simulink model "ITCG_3D"  (R2023b)
settings: Solver=FixedStepAuto  StartTime=0.0  StopTime=45  FixedStep=1/100  RelTol=1e-3
libraries: simulink x1
settings Model: NumberOfSteps=10  PacingRate=5  Creator=Administrator  LastModifiedBy=lmj04
settings DebuggingCC: UnderSpecifiedDimensionMsg=warning

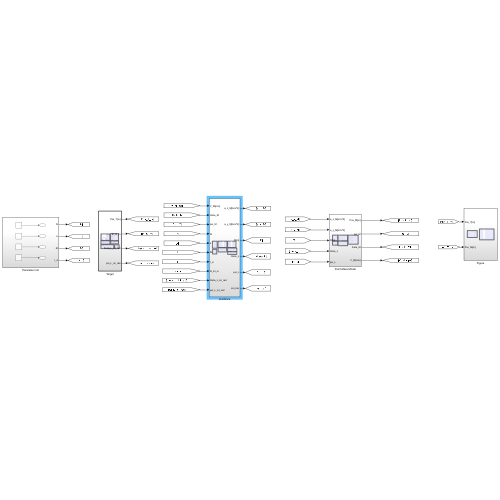
[thumbnail: Simulink's stored preview of the top-level diagram]
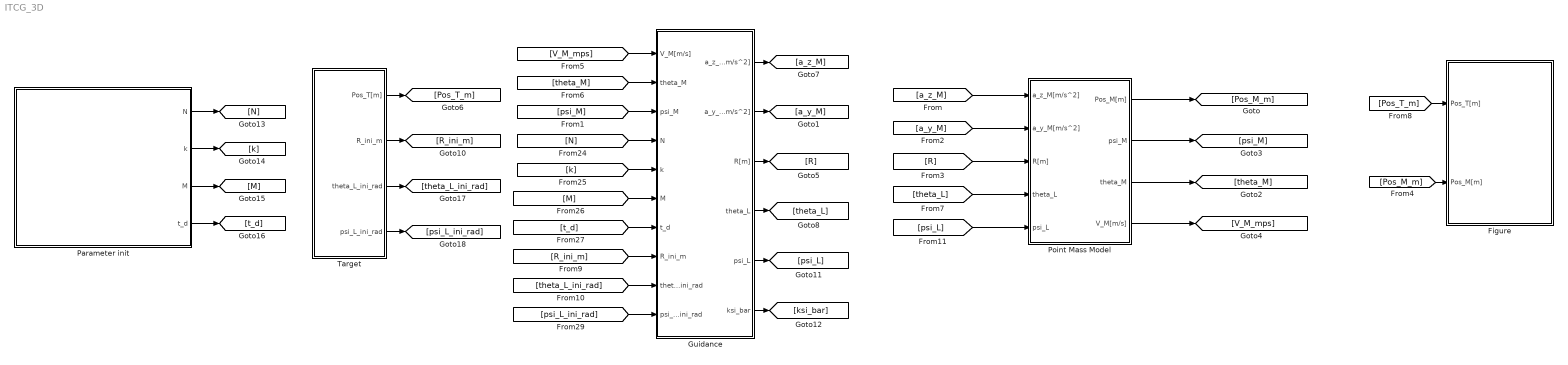
== system ITCG_3D ==
  Figure : Subsystem
  Guidance : Subsystem
  Parameter init : Subsystem
  Point Mass Model : Subsystem
  Target : Subsystem  TreatAsAtomicUnit=on
  wires:
  Target/1(Pos_T[m]) -> [Pos_T_m]
  Guidance/1(a_z_M[m/s^2]) -> [a_z_M]
  [V_M_mps] -> Guidance/1(V_M[m/s])
  Point Mass Model/1(Pos_M[m]) -> [Pos_M_m]
  Point Mass Model/4(V_M[m/s]) -> [V_M_mps]
  Guidance/2(a_y_M[m/s^2]) -> [a_y_M]
  Guidance/3(R[m]) -> [R]
  [R] -> Point Mass Model/3(R[m])
  Guidance/4(theta_L) -> [theta_L]
  [theta_L] -> Point Mass Model/4(theta_L)
  Point Mass Model/2(psi_M) -> [psi_M]
  Point Mass Model/3(theta_M) -> [theta_M]
  [theta_M] -> Guidance/2(theta_M)
  [psi_M] -> Guidance/3(psi_M)
  Guidance/5(psi_L) -> [psi_L]
  [psi_L] -> Point Mass Model/5(psi_L)
  Guidance/6(ksi_bar) -> [ksi_bar]
  Parameter init/2(k) -> [k]
  Parameter init/1(N) -> [N]
  Parameter init/3(M) -> [M]
  Parameter init/4(t_d) -> [t_d]
  [M] -> Guidance/6(M)
  [t_d] -> Guidance/7(t_d)
  [N] -> Guidance/4(N)
  [k] -> Guidance/5(k)
  [a_y_M] -> Point Mass Model/2(a_y_M[m/s^2])
  Target/2(R_ini_m) -> [R_ini_m]
  [R_ini_m] -> Guidance/8(R_ini_m)
  Target/3(theta_L_ini_rad) -> [theta_L_ini_rad]
  Target/4(psi_L_ini_rad) -> [psi_L_ini_rad]
  [theta_L_ini_rad] -> Guidance/9(theta_L_ini_rad)
  [psi_L_ini_rad] -> Guidance/10(psi_L_ini_rad)
  [a_z_M] -> Point Mass Model/1(a_z_M[m/s^2])
  [Pos_M_m] -> Figure/2(Pos_M[m])
  [Pos_T_m] -> Figure/1(Pos_T[m])

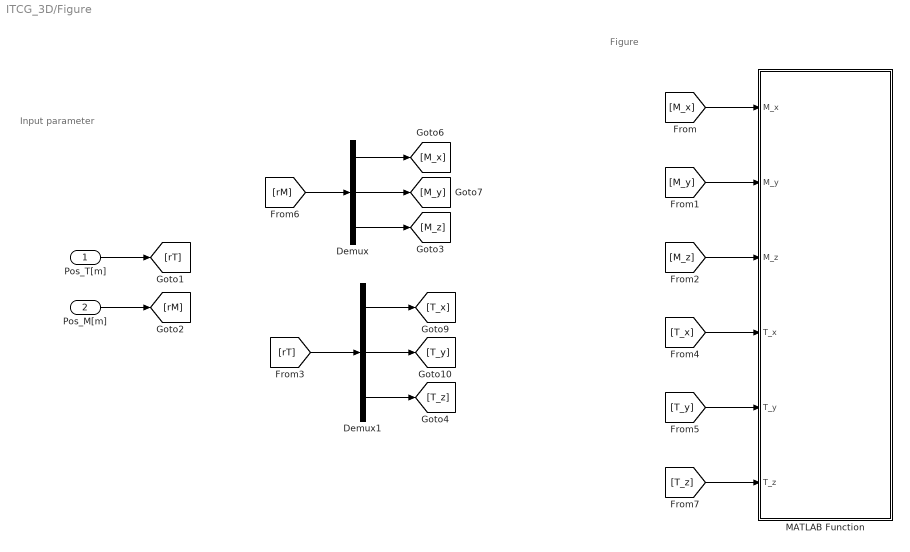
== system ITCG_3D/Figure ==
  note: Figure
  note: Input parameter
  Pos_T[m] : Inport
  Pos_M[m] : Inport  Port=2
  Demux : Demux  Outputs=3
  Demux1 : Demux  Outputs=3
  MATLAB Function : MATLAB Function  TreatAsAtomicUnit=on
  wires:
  Pos_T[m]/1 -> [rT]
  Pos_M[m]/1 -> [rM]
  [rT] -> Demux1/1
  Demux1/1 -> [T_x]
  Demux1/2 -> [T_y]
  Demux/2 -> [M_y]
  Demux/1 -> [M_x]
  Demux/3 -> [M_z]
  Demux1/3 -> [T_z]
  [M_x] -> MATLAB Function/1(M_x)
  [M_y] -> MATLAB Function/2(M_y)
  [M_z] -> MATLAB Function/3(M_z)
  [T_x] -> MATLAB Function/4(T_x)
  [T_y] -> MATLAB Function/5(T_y)
  [T_z] -> MATLAB Function/6(T_z)
  [rM] -> Demux/1

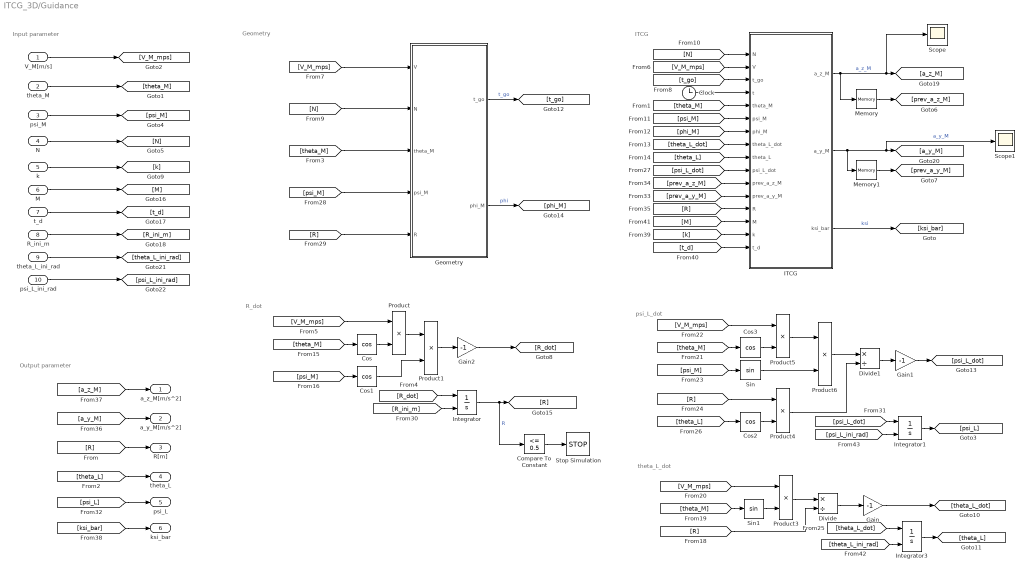
== system ITCG_3D/Guidance ==
  note: ITCG
  note: Geometry
  note: Input parameter
  note: Output parameter
  note: psi_L_dot
  note: theta_L_dot
  note: R_dot
  V_M[m/s] : Inport
  theta_M : Inport  Port=2
  psi_M : Inport  Port=3
  N : Inport  Port=4
  k : Inport  Port=5
  M : Inport  Port=6
  t_d : Inport  Port=7
  R_ini_m : Inport  Port=8
  theta_L_ini_rad : Inport  Port=9
  psi_L_ini_rad : Inport  Port=10
  Clock : Clock
  Compare To Constant : simulink/Logic and Bit Operations/Compare To Constant  relop=<=  const=0.5  OutDataTypeStr=boolean
  Cos{,1..3} (4 alike) : Trigonometry  Operator=cos
  Divide : Product  Inputs=*/
  Divide1 : Product  Inputs=*/
  Gain : Gain  Gain=-1
  Gain1 : Gain  Gain=-1
  Gain2 : Gain  Gain=-1
  Geometry : MATLAB Function  TreatAsAtomicUnit=on
  ITCG : MATLAB Function  TreatAsAtomicUnit=on
  Integrator : Integrator  InitialConditionSource=external  InitialCondition=sqrt(300^2+500^2)
  Integrator1 : Integrator  InitialConditionSource=external
  Integrator3 : Integrator  InitialConditionSource=external
  Memory : Memory
  Memory1 : Memory
  Product{,1,3..6} (6 alike) : Product
  Scope : Scope
  Scope1 : Scope
  Sin : Trigonometry
  Sin1 : Trigonometry
  Stop Simulation : Stop
  a_z_M[m/s^2] : Outport
  a_y_M[m/s^2] : Outport  Port=2
  R[m] : Outport  Port=3
  theta_L : Outport  Port=4
  psi_L : Outport  Port=5
  ksi_bar : Outport  Port=6
  wires:
  V_M[m/s]/1 -> [V_M_mps]
  [V_M_mps] -> Geometry/1(V)
  N/1 -> [N]
  [N] -> Geometry/2(N)
  ITCG/3(ksi_bar) -> [ksi_bar]  "ksi"
  [N] -> ITCG/1(N)
  [V_M_mps] -> ITCG/2(V)
  [t_go] -> ITCG/3(t_go)
  Clock/1 -> ITCG/4(t)
  [theta_M] -> ITCG/5(theta_M)
  [psi_M] -> ITCG/6(psi_M)
  [phi_M] -> ITCG/7(phi_M)
  [theta_L_dot] -> ITCG/8(theta_L_dot)
  [theta_L] -> ITCG/9(theta_L)
  theta_M/1 -> [theta_M]
  psi_M/1 -> [psi_M]
  [V_M_mps] -> Product/1
  Cos/1 -> Product/2
  [theta_M] -> Cos/1
  Product/1 -> Product1/1
  [psi_M] -> Cos1/1
  Cos1/1 -> Product1/2
  Gain2/1 -> [R_dot]
  Sin1/1 -> Product3/2
  [V_M_mps] -> Product3/1
  [theta_M] -> Sin1/1
  Product3/1 -> Divide/1
  [R] -> Divide/2
  Divide/1 -> Gain/1
  [theta_M] -> Cos3/1
  [V_M_mps] -> Product5/1
  Cos3/1 -> Product5/2
  Product5/1 -> Product6/1
  [psi_M] -> Sin/1
  Sin/1 -> Product6/2
  [theta_L_dot] -> Integrator3/1
  Integrator3/1 -> [theta_L]
  Product6/1 -> Divide1/1
  Divide1/1 -> Gain1/1
  Geometry/1(t_go) -> [t_go]  "t_go"
  Geometry/2(phi_M) -> [phi_M]  "phi"
  [theta_M] -> Geometry/3(theta_M)
  [theta_L] -> theta_L/1
  [R] -> R[m]/1
  [psi_M] -> Geometry/4(psi_M)
  [psi_L_dot] -> ITCG/10(psi_L_dot)
  [R_dot] -> Integrator/1
  [a_y_M] -> a_y_M[m/s^2]/1
  [a_z_M] -> a_z_M[m/s^2]/1
  ITCG/1(a_z_M) -> Scope/1, [a_z_M], Memory/1  "a_z_M"
  ITCG/2(a_y_M) -> Memory1/1, Scope1/1, [a_y_M]  "a_y_M"
  Gain/1 -> [theta_L_dot]
  Gain1/1 -> [psi_L_dot]
  Integrator/1 -> [R], Compare To Constant/1  "R"
  [R] -> Product4/1
  Cos2/1 -> Product4/2
  [theta_L] -> Cos2/1
  Product4/1 -> Divide1/2
  Product1/1 -> Gain2/1
  [R] -> Geometry/5(R)
  [psi_L_dot] -> Integrator1/1
  Integrator1/1 -> [psi_L]
  [psi_L] -> psi_L/1
  Memory/1 -> [prev_a_z_M]
  Memory1/1 -> [prev_a_y_M]
  [prev_a_y_M] -> ITCG/12(prev_a_y_M)
  [prev_a_z_M] -> ITCG/11(prev_a_z_M)
  [R] -> ITCG/13(R)
  [ksi_bar] -> ksi_bar/1
  k/1 -> [k]
  M/1 -> [M]
  t_d/1 -> [t_d]
  [M] -> ITCG/14(M)
  [k] -> ITCG/15(k)
  [t_d] -> ITCG/16(t_d)
  Compare To Constant/1 -> Stop Simulation/1
  R_ini_m/1 -> [R_ini_m]
  [R_ini_m] -> Integrator/2
  theta_L_ini_rad/1 -> [theta_L_ini_rad]
  psi_L_ini_rad/1 -> [psi_L_ini_rad]
  [theta_L_ini_rad] -> Integrator3/2
  [psi_L_ini_rad] -> Integrator1/2

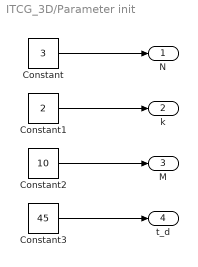
== system ITCG_3D/Parameter init ==
  Constant : Constant  Value=3
  Constant1 : Constant  Value=2
  Constant2 : Constant  Value=10
  Constant3 : Constant  Value=45
  N : Outport
  k : Outport  Port=2
  M : Outport  Port=3
  t_d : Outport  Port=4
  wires:
  Constant/1 -> N/1
  Constant1/1 -> k/1
  Constant2/1 -> M/1
  Constant3/1 -> t_d/1

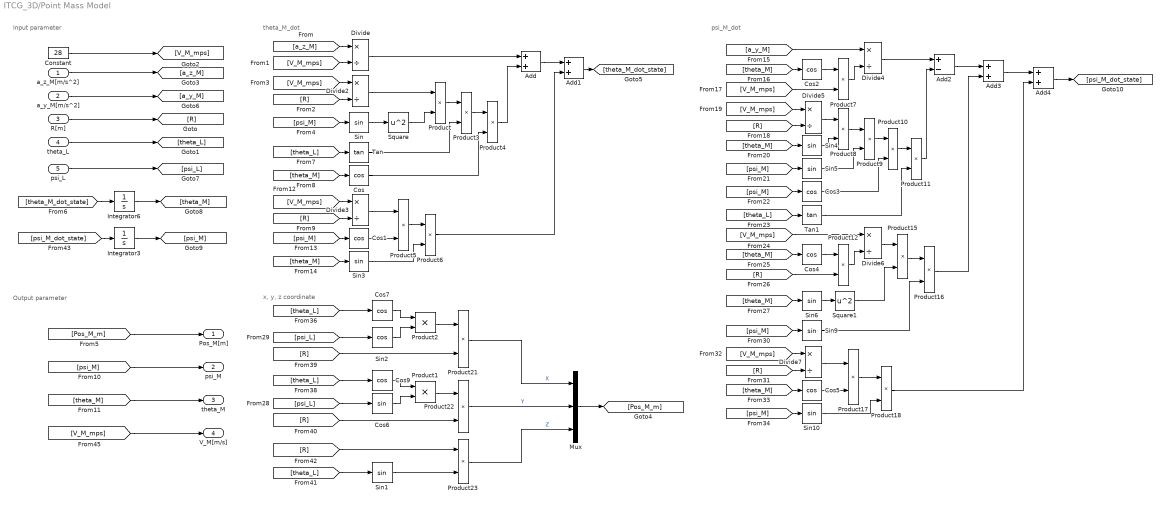
== system ITCG_3D/Point Mass Model ==
  note: Output parameter
  note: Input parameter
  note: theta_M_dot
  note: x, y, z coordinate
  note: psi_M_dot
  a_z_M[m/s^2] : Inport
  a_y_M[m/s^2] : Inport  Port=2
  R[m] : Inport  Port=3
  theta_L : Inport  Port=4
  psi_L : Inport  Port=5
  Add{,1,3..4} (4 alike) : Sum
  Add2 : Sum  Inputs=+-
  Constant : Constant  Value=28
  Cos{,1..5,7,9} (8 alike) : Trigonometry  Operator=cos
  Cos6 : Trigonometry
  Divide{,2..7} (7 alike) : Product  Inputs=*/
  Integrator3 : Integrator  InitialCondition=10*pi/180
  Integrator6 : Integrator  InitialCondition=10*pi/180
  Mux : Mux  Inputs=3
  Product{,1..12,15..18,21..23} (20 alike) : Product
  Sin{,1,3..6,9..10} (8 alike) : Trigonometry
  Sin2 : Trigonometry  Operator=cos
  Square : Math  Operator=square
  Square1 : Math  Operator=square
  Tan : Trigonometry  Operator=tan
  Tan1 : Trigonometry  Operator=tan
  Pos_M[m] : Outport
  psi_M : Outport  Port=2
  theta_M : Outport  Port=3
  V_M[m/s] : Outport  Port=4
  wires:
  Constant/1 -> [V_M_mps]
  a_z_M[m/s^2]/1 -> [a_z_M]
  a_y_M[m/s^2]/1 -> [a_y_M]
  [a_z_M] -> Divide/1
  [V_M_mps] -> Divide/2
  Divide/1 -> Add/1
  [V_M_mps] -> Divide2/1
  R[m]/1 -> [R]
  theta_L/1 -> [theta_L]
  [R] -> Divide2/2
  Divide2/1 -> Product/1
  [psi_M] -> Sin/1
  Sin/1 -> Square/1
  Square/1 -> Product/2
  [theta_L] -> Tan/1
  Product/1 -> Product3/1
  Tan/1 -> Product3/2
  [theta_M] -> Cos/1
  Product3/1 -> Product4/1
  Cos/1 -> Product4/2
  Product4/1 -> Add/2
  [V_M_mps] -> Divide3/1
  [R] -> Divide3/2
  Divide3/1 -> Product5/1
  [psi_M] -> Cos1/1
  Cos1/1 -> Product5/2
  Product5/1 -> Product6/1
  [theta_M] -> Sin3/1
  Sin3/1 -> Product6/2
  Add/1 -> Add1/1
  Product6/1 -> Add1/2
  Add1/1 -> [theta_M_dot_state]
  [a_y_M] -> Divide4/1
  [theta_M] -> Cos2/1
  Cos2/1 -> Product7/1
  [V_M_mps] -> Product7/2
  Product7/1 -> Divide4/2
  Divide4/1 -> Add2/1
  [V_M_mps] -> Divide5/1
  [R] -> Divide5/2
  Divide5/1 -> Product8/1
  [theta_M] -> Sin4/1
  Sin4/1 -> Product8/2
  [psi_M] -> Sin5/1
  Product8/1 -> Product9/1
  Sin5/1 -> Product9/2
  [psi_M] -> Cos3/1
  Product9/1 -> Product10/1
  Cos3/1 -> Product10/2
  [theta_L] -> Tan1/1
  Product10/1 -> Product11/1
  Tan1/1 -> Product11/2
  Product11/1 -> Add2/2
  [R] -> Product12/2
  Product12/1 -> Divide6/2
  [V_M_mps] -> Divide6/1
  Cos4/1 -> Product12/1
  [theta_M] -> Cos4/1
  [theta_M] -> Sin6/1
  Sin6/1 -> Square1/1
  [psi_M] -> Sin9/1
  Square1/1 -> Product15/2
  Sin9/1 -> Product16/2
  Divide6/1 -> Product15/1
  Product15/1 -> Product16/1
  Add2/1 -> Add3/1
  Product16/1 -> Add3/2
  Add3/1 -> Add4/1
  [V_M_mps] -> Divide7/1
  [R] -> Divide7/2
  Divide7/1 -> Product17/1
  [theta_M] -> Cos5/1
  Cos5/1 -> Product17/2
  [psi_M] -> Sin10/1
  Product17/1 -> Product18/1
  Sin10/1 -> Product18/2
  Product18/1 -> Add4/2
  Add4/1 -> [psi_M_dot_state]
  [theta_L] -> Cos7/1
  [theta_L] -> Cos9/1
  [R] -> Product21/2
  [R] -> Product22/2
  [theta_L] -> Sin1/1
  [R] -> Product23/1
  Sin1/1 -> Product23/2
  [psi_M_dot_state] -> Integrator3/1
  [V_M_mps] -> V_M[m/s]/1
  [Pos_M_m] -> Pos_M[m]/1
  [psi_M] -> psi_M/1
  [theta_M] -> theta_M/1
  [theta_M_dot_state] -> Integrator6/1
  Integrator6/1 -> [theta_M]
  Integrator3/1 -> [psi_M]
  Cos9/1 -> Product1/1
  Product1/1 -> Product22/1
  [psi_L] -> Cos6/1
  Cos6/1 -> Product1/2
  Cos7/1 -> Product2/1
  Product2/1 -> Product21/1
  [psi_L] -> Sin2/1
  Sin2/1 -> Product2/2
  psi_L/1 -> [psi_L]
  Mux/1 -> [Pos_M_m]
  Product21/1 -> Mux/1  "X"
  Product22/1 -> Mux/2  "Y"
  Product23/1 -> Mux/3  "Z"

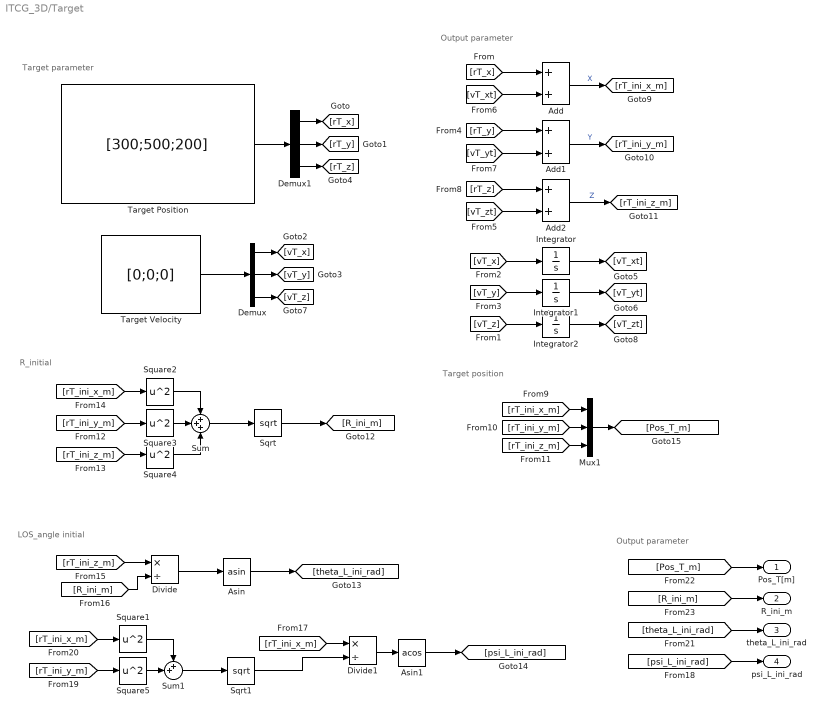
== system ITCG_3D/Target ==
  note: Output parameter
  note: Target position
  note: LOS_angle initial
  note: R_initial
  note: Output parameter
  note: Target parameter
  Add : Sum
  Add1 : Sum
  Add2 : Sum
  Asin : Trigonometry  Operator=asin
  Asin1 : Trigonometry  Operator=acos
  Demux : Demux  Outputs=3
  Demux1 : Demux  Outputs=3
  Divide : Product  Inputs=*/
  Divide1 : Product  Inputs=*/
  Integrator : Integrator
  Integrator1 : Integrator
  Integrator2 : Integrator
  Mux1 : Mux  Inputs=3
  Sqrt : Sqrt
  Sqrt1 : Sqrt
  Square{1..5} (5 alike) : Math  Operator=square
  Sum : Sum  Inputs=+++
  Sum1 : Sum  Inputs=++|
  Target Position : Constant  Value=[300;500;200]  VectorParams1D=off
  Target Velocity : Constant  Value=[0;0;0]  VectorParams1D=off
  Pos_T[m] : Outport
  R_ini_m : Outport  Port=2
  theta_L_ini_rad : Outport  Port=3
  psi_L_ini_rad : Outport  Port=4
  wires:
  Target Velocity/1 -> Demux/1
  Target Position/1 -> Demux1/1
  Add/1 -> [rT_ini_x_m]  "X"
  Add1/1 -> [rT_ini_y_m]  "Y"
  Demux1/1 -> [rT_x]
  [rT_x] -> Add/1
  Demux1/2 -> [rT_y]
  [rT_y] -> Add1/1
  Demux/1 -> [vT_x]
  Demux/2 -> [vT_y]
  [vT_xt] -> Add/2
  [vT_yt] -> Add1/2
  [vT_x] -> Integrator/1
  [vT_y] -> Integrator1/1
  Integrator/1 -> [vT_xt]
  Integrator1/1 -> [vT_yt]
  Demux1/3 -> [rT_z]
  Demux/3 -> [vT_z]
  [vT_z] -> Integrator2/1
  Integrator2/1 -> [vT_zt]
  [vT_zt] -> Add2/2
  [rT_z] -> Add2/1
  Add2/1 -> [rT_ini_z_m]  "Z"
  Sum/1 -> Sqrt/1
  Sqrt/1 -> [R_ini_m]
  Square2/1 -> Sum/1
  Square4/1 -> Sum/3
  Square3/1 -> Sum/2
  [rT_ini_x_m] -> Mux1/1
  [rT_ini_y_m] -> Mux1/2
  [rT_ini_z_m] -> Mux1/3
  [rT_ini_x_m] -> Square2/1
  [rT_ini_y_m] -> Square3/1
  [rT_ini_z_m] -> Square4/1
  [rT_ini_z_m] -> Divide/1
  [R_ini_m] -> Divide/2
  Divide/1 -> Asin/1
  Sqrt1/1 -> Divide1/2
  [rT_ini_x_m] -> Divide1/1
  Divide1/1 -> Asin1/1
  [rT_ini_y_m] -> Square5/1
  [rT_ini_x_m] -> Square1/1
  Square5/1 -> Sum1/2
  Square1/1 -> Sum1/1
  Sum1/1 -> Sqrt1/1
  Asin/1 -> [theta_L_ini_rad]
  Asin1/1 -> [psi_L_ini_rad]
  Mux1/1 -> [Pos_T_m]
  [psi_L_ini_rad] -> psi_L_ini_rad/1
  [theta_L_ini_rad] -> theta_L_ini_rad/1
  [Pos_T_m] -> Pos_T[m]/1
  [R_ini_m] -> R_ini_m/1

== matlab function ITCG_3D/Guidance/Geometry ==
  data: V input; N input; t_go output; phi_M output; theta_M input; psi_M input; R input
function [t_go, phi_M] =fcn(V, N, theta_M, psi_M, R)
    D2R=pi/180;

    phi_M=acos(cos(theta_M)*cos(psi_M));

    % if abs(phi_M) < 3*D2R
    %     phi_M=1e-3;
    % end

    %% t_go calculate
    a = 1 / (2 * (N - 1));
    b = 1 / 2;
    B1 = integral(@(t) t.^(a-1) .* (1-t).^(b-1), 0, sin(phi_M)^2, "AbsTol", 1e-6, "RelTol", 1e-4);
    B2 = integral(@(t) t.^(a-1) .* (1-t).^(b-1), 0, 1, "AbsTol", 1e-6, "RelTol", 1e-4);
% B1 = integral(@(t) t.^(a-1) .* (1-t).^(b-1), 0, sin(phi_M)^2);
%     B2 = integral(@(t) t.^(a-1) .* (1-t).^(b-1), 0, 1);
    % B2 = beta(a, b);

    % if isnan(B1)
    %     B1 = 0;
    % end
    % if isnan(B2)
    %     B2 = 0;
    % end

    if abs(phi_M) >= 0 && abs(phi_M) < pi / 2
        t_go = (R  / (2 * V * (N-1) * sin(phi_M)^(1 / (N-1) ) ) ) * B1;
        if isinf(t_go)
            t_go = 0;
        end

    else
        t_go = (R / (2 * V  * (N-1) * sin(phi_M)^(1 / (N-1) ) ) ) * (2 * B2 - B1);
        if isinf(t_go)
            t_go = 0;
        end
    end

    % t_go=(R / V) * (1 + (phi_M^2 / ( 2 * (2 * N - 1) ) ) );

    % theta_L_dot=-V*sin(theta_M)/R;
    % if theta_L_dot >=0
    %     theta_L_dot=0;
    % end
    % psi_L_dot=-V*cos(theta_M)*sin(psi_M)/(R*cos(theta_L));
    % if psi_L_dot >=0
    %     psi_L_dot=0;
    % end

== matlab function ITCG_3D/Figure/MATLAB Function ==
  settings: updateMethod=DISCRETE
  data: M_x input; M_y input; M_z input; T_x input; T_y input; T_z input
function fcn(M_x, M_y, M_z, T_x, T_y, T_z)

persistent data timeldx data2 data3 

if isempty(data)      
    data=zeros(100000,3);
    timeldx=1;
end

if isempty(data2)
    data2=zeros(100000,3);
    timeldx=1;
end

if isempty(data3)
    data3=zeros(100000,3);
    timeldx=1;
end

pos_missile=zeros(1,3);
pos_missile(1,1)=M_x;
pos_missile(1,2)=M_y;
pos_missile(1,3)=M_z;


pos_target=zeros(1,3);
pos_target(1,1)=T_x;
pos_target(1,2)=T_y;
pos_target(1,3)=T_z;

R=zeros(1,1);
R(1,1)=sqrt((T_x-M_x)^2+(T_y-M_y)^2+(T_z-M_z)^2);

data(timeldx,:)=pos_missile;
data2(timeldx,:)=pos_target;
data3(timeldx,:)=R;



plot3(data(1:timeldx,1), data(1:timeldx,2), data(1:timeldx, 3));
grid;
hold on;
plot3(0,0, 00, '*');

plot3(M_x, M_y, M_z, 'rpentagram', 'LineWidth',1);

plot3(data(1:timeldx,1), data(1:timeldx,2), data(1:timeldx,3));
plot3(data2(1:timeldx,1), data2(1:timeldx,2), data2(1:timeldx,3),'*');

title('Impact Time Control Guidance')
xlabel('X(m)')
ylabel('Y(m)')
zlabel('Z(m)')
hold off;

timeldx=timeldx+1;

end

== matlab function ITCG_3D/Guidance/ITCG ==
  data: a_z_M output; a_y_M output; N input; V input; t_go input; t input; theta_M input; ksi_bar output; psi_M input; phi_M input; theta_L_dot input; theta_L input; psi_L_dot input; prev_a_z_M input; prev_a_y_M input; R input; M input; k input; t_d input
function [a_z_M, a_y_M, ksi_bar]  = fcn(N, V, t_go, t, theta_M, psi_M, phi_M, theta_L_dot, theta_L, psi_L_dot, prev_a_z_M, prev_a_y_M, R, M, k, t_d)
    
    ksi_bar=t_go-t_d+t;
    % 
    % if ksi_bar>-0.1
    %     ksi_bar=0;
    % end
    sgmf_ksi_bar = 2 * ( (1 / ( 1 + exp( -10 * ksi_bar ) ) ) - 1 / 2 );
    sgmf_phi_M= 2 * ( ( 1 / ( 1 + exp( -10 * abs(phi_M) ) ) ) - 1 / 2);
    %% ITCG command
    if t<30
        a_y_M = -N * (1 + k * sgmf_ksi_bar) * V * ((-theta_L_dot * sin(theta_M) * sin(psi_M)) - (psi_L_dot * cos(theta_L) * cos(theta_M))) + M * (sgmf_phi_M - 1) * sgmf_ksi_bar*1;
        a_z_M = 0;
    else
        a_y_M = -N * (1 + k * sgmf_ksi_bar) * V * ((-theta_L_dot * sin(theta_M) * sin(psi_M)) - (psi_L_dot * cos(theta_L) * cos(theta_M))) + M * (sgmf_phi_M - 1) * sgmf_ksi_bar*1;
        a_z_M = N * (1 + k * sgmf_ksi_bar) * (V * theta_L_dot * cos(psi_M)) + M * (sgmf_phi_M - 1) * sgmf_ksi_bar*1;    %% ITCG command
    end

    % if R<10
    %     a_y_M=prev_a_y_M;
    %     a_z_M=prev_a_z_M;
    % else
    %     a_y_M = -N * (1 + k * sgmf_ksi_bar) * V * ((-theta_L_dot * sin(theta_M) * sin(psi_M)) - (psi_L_dot * cos(theta_L) * cos(theta_M))) + M * (sgmf_phi_M - 1) * sgmf_ksi_bar*1;
    %     a_z_M = N * (1 + k * sgmf_ksi_bar) * (V * theta_L_dot * cos(psi_M)) + M * (sgmf_phi_M - 1) * sgmf_ksi_bar*1;
    % end
